simulink model "Lesson_1"  (R2022b)
settings: Solver=VariableStepAuto  StartTime=0.0  StopTime=0.06  RelTol=1e-3
values from neighbouring files (symbols this model uses):
  L = 0.004    [Lesson_1.m]
  R = 5    [Lesson_1.m]
settings Model: Creator=adlercohen  LastModifiedBy=adlercohen

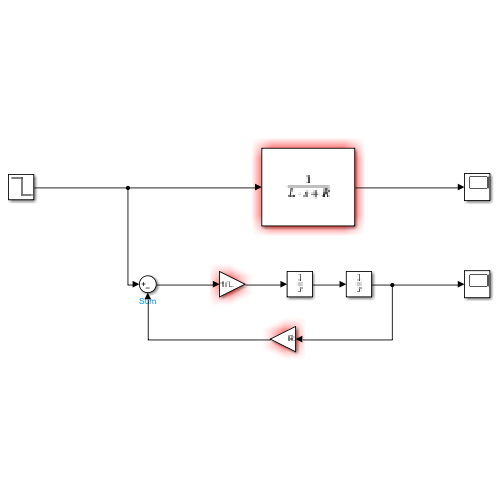
[thumbnail: Simulink's stored preview of the top-level diagram]
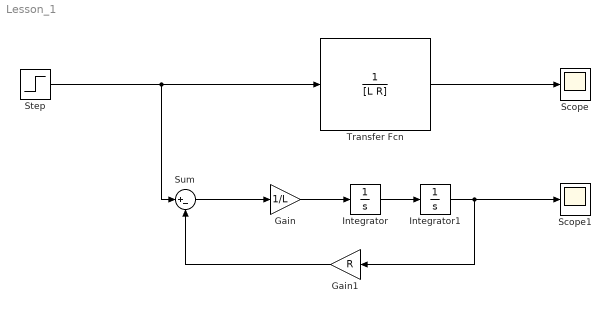
== system Lesson_1 ==
  Gain : Gain  Gain=1/L
  Gain1 : Gain  Gain=R
  Integrator : Integrator
  Integrator1 : Integrator
  Scope : Scope
  Scope1 : Scope
  Step : Step  Time=0  Before=10  SampleTime=0
  Sum : Sum  Inputs=|+-
  Transfer Fcn : TransferFcn  Denominator=[L R]
  wires:
  Step/1 -> Transfer Fcn/1, Sum/1
  Transfer Fcn/1 -> Scope/1
  Integrator/1 -> Integrator1/1
  Gain1/1 -> Sum/2
  Sum/1 -> Gain/1
  Gain/1 -> Integrator/1
  Integrator1/1 -> Gain1/1, Scope1/1
